simulink model "RotorTune_ver3f"  (R2024a)
settings: Solver=FixedStepAuto  StartTime=0.0  StopTime=Inf  FixedStep=SampleTs  RelTol=1e-3  EnableMultiTasking=on
values from neighbouring files (symbols this model uses):
  A = [0, 1 ... (first row only)    [linearisze_lqr_design.m]
undefined symbols (not defined in the file or in its folder): ControlTs, ctrlDen, ctrlNum, Den, Down, EncBias, EncRes, fdbkctrl, fdbkopt, GPTRIP1SEL, Num, SampleTs, SimTime, StartTime, StepMagnitude, T_L, TZ1, Up, VelRes
libraries: simulink x3, c2837xDlib x1, c2802xlib x1, c280xlib x1
settings Model: SimulationMode=external  ExtModeTrigDuration=8  Creator=Student  LastModifiedBy=MAELAB_05
settings OptimizationCC: DefaultUnderspecifiedDataType=single  EnhancedBackFolding=on  PassReuseOutputArgsAs=Individual arguments  MaxStackSize=1024  OptimizeBlockOrder=speed  DifferentSizesBufferReuse=on  OptimizationCustomize=off  DenormalBehavior=FlushToZero  EfficientTunableParamExpr=on
settings DebuggingCC: ParameterTunabilityLossMsg=error
settings HardwareCC: ProdBitPerChar=16  ProdBitPerInt=16  ProdBitPerPointer=32  ProdBitPerSizeT=32  ProdBitPerPtrDiffT=32  ProdLargestAtomicInteger=Integer  ProdLargestAtomicFloat=None  ProdWordSize=16  ProdLongLongMode=on  ProdHWDeviceType=Texas Instruments->C2000
settings ModelReferenceCC: ModelReferenceNumInstancesAllowed=Single
settings SFSimCC: MATLABDynamicMemAlloc=off
settings RTWCC: Description=Embedded Coder  SystemTargetFile=ert.tlc  HardwareBoard=TI Delfino F28379D LaunchPad  TemplateMakefile=ert_default_tmf  Toolchain=Texas Instruments Code Composer Studio (C2000)  CodeProfilingSaveOptions=MetricsOnly  GPUComputeCapability=3.5
settings CodeAppCC: ForceParamTrailComments=on  IgnoreCustomStorageClasses=off  OperatorAnnotations=on  SimulinkDataObjDesc=on  SFDataObjDesc=on  InsertBlockDesc=on
settings ERTTargetCC: CodeReplacementLibrary=TI C28x  ExtMode=on  ExtModeTransport=4  ExtModeStaticAlloc=on  ExtModeAutomaticAllocSize=off  ExtModeStaticAllocSize=10000  ExtModeMexFile=ext_xcp  ExtModeMexArgs=1 4 5000000  ExtModeIntrfLevel=Level2 - Open

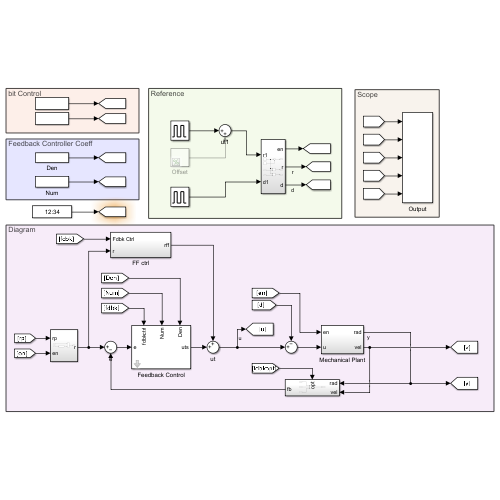
[thumbnail: Simulink's stored preview of the top-level diagram]
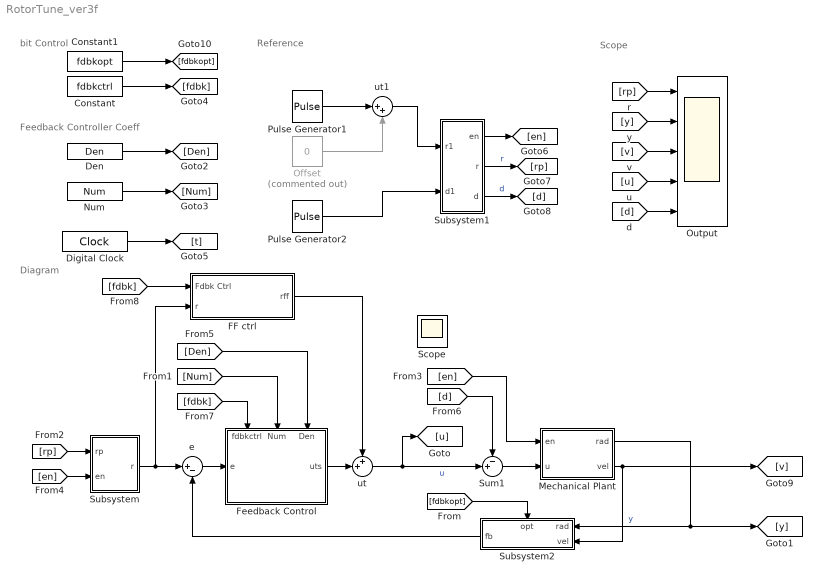
== system RotorTune_ver3f ==
  note: Diagram
  note: Scope
  note: Reference
  note: bit Control
  note: Feedback Controller Coeff
  Constant : Constant  Value=fdbkctrl  OutDataTypeStr=double  SampleTime=SampleTs
  Constant1 : Constant  Value=fdbkopt  OutDataTypeStr=double  SampleTime=SampleTs
  Den : Constant  Value=Den  SampleTime=ControlTs
  Digital Clock : DigitalClock  SampleTime=SampleTs
  FF ctrl : Subsystem
  Feedback Control : Subsystem  mask(Discrete Time Controller){}
      mask help: Discrete IIR filter with output saturation. Please write the controller in filter form before writing the numerator and denominator coefficients.
      settings: PortSchema="{\"entries\":[{\"content\":{\"sides\":[{\"content\":{\"connectorIds\":[\"In1\"]},\"type\":\"ConnectorPlacement.EquallySpacedRectSide\",\"uuid\":\"e0eb88a8-3f62-4736-a83e-fbf139955186\"},{\"content\":{\"connectorIds\":[\"Out1\"],\"side\":\"RIGHT\"},\"type\":\"ConnectorPlacement.EquallySpacedRectSide\",\"uuid\":\"655529f7-d729-4d0c-b17c-6f52c7004a6d\"},{\"content\":{\"connectorIds\":[\"In2\",\"In3\",\"In4\"],\"side\":\"TOP\"},\"type\":\"ConnectorPlacement.EquallySpacedRectSide\",\"uuid\":\"a879eb77-4166-453f-a794-1fc287420031\"},{\"content\":{\"connectorIds\":[],\"side\":\"BOTTOM\"},\"type\":\"ConnectorPlacement.EquallySpacedRectSide\",\"uuid\":\"f5f0df5c-bd43-42ec-91f5-1b4d11260522\"}]},\"type\":\"ConnectorPlacement.EquallySpacedConnector\",\"uuid\":\"5f5b86c4-0571-4a61-ae4f-21c2576f152a\"}],\"packageUris\":[\"http://schema.mathworks.com/mf0/Connector/R2020b\"],\"version\":\"1.0\"}"
  Mechanical Plant : Subsystem
  Num : Constant  Value=Num  SampleTime=ControlTs
  Offset : Constant  Commented=on  Value=0
  Output : Scope  NumInputPorts=5
  Pulse Generator1 : DiscretePulseGenerator  PulseType=Time based  Amplitude=StepMagnitude  Period=10  PulseWidth=50
  Pulse Generator2 : DiscretePulseGenerator  PulseType=Time based  Amplitude=T_L*fdbkctrl  Period=10  PulseWidth=50  PhaseDelay=1
  Subsystem : Subsystem
  Subsystem1 : Subsystem
  Subsystem2 : Subsystem
      settings: PortSchema="{\"entries\":[{\"content\":{\"sides\":[{\"content\":{\"connectorIds\":[\"Out1\"]},\"type\":\"ConnectorPlacement.EquallySpacedRectSide\",\"uuid\":\"4f8a58ab-8b77-4548-a5e4-8c342b5af4de\"},{\"content\":{\"connectorIds\":[\"In2\",\"In3\"],\"side\":\"RIGHT\"},\"type\":\"ConnectorPlacement.EquallySpacedRectSide\",\"uuid\":\"f569d0f3-df36-4b5a-9df6-29756aab0033\"},{\"content\":{\"connectorIds\":[\"In1\"],\"side\":\"TOP\"},\"type\":\"ConnectorPlacement.EquallySpacedRectSide\",\"uuid\":\"c4523680-dffb-4dca-b5af-4725fc2c115b\"}]},\"type\":\"ConnectorPlacement.EquallySpacedConnector\",\"uuid\":\"6d4037b4-5141-4a52-bd71-8d22041459e1\"}],\"packageUris\":[\"http://schema.mathworks.com/mf0/Connector/R2020b\"],\"version\":\"1.0\"}"
  Sum1 : Sum  Inputs=-+|
  e : Sum  Inputs=|+-
  ut : Sum  Inputs=++|
  ut1 : Sum  Inputs=|++
  Scope : Scope
  wires:
  [en] -> Mechanical Plant/1(en)
  Feedback Control/1(uts) -> ut/2
  [rp] -> Subsystem/1(rp)
  [en] -> Subsystem/2(en)
  Subsystem/1(r) -> e/1, FF ctrl/2(r)
  FF ctrl/1(rff) -> ut/1
  e/1 -> Feedback Control/1(e)
  [fdbk] -> Feedback Control/2(fdbkctrl)
  Den/1 -> [Den]
  Num/1 -> [Num]
  [Den] -> Feedback Control/4(Den)
  Constant/1 -> [fdbk]
  ut/1 -> Sum1/2, [u]  "u"
  [d] -> Sum1/1
  Sum1/1 -> Mechanical Plant/2(u)
  Subsystem1/1(en) -> [en]
  Subsystem1/2(r) -> [rp]  "r"
  Subsystem1/3(d) -> [d]  "d"
  [rp] -> Output/1
  [y] -> Output/2
  Mechanical Plant/2(vel) -> Subsystem2/3(vel), [v]
  [v] -> Output/3
  [u] -> Output/4
  [d] -> Output/5
  ut1/1 -> Subsystem1/1(r1)
  Pulse Generator1/1 -> ut1/1
  Offset/1 -> ut1/2
  Digital Clock/1 -> [t]
  [Num] -> Feedback Control/3(Num)
  [fdbk] -> FF ctrl/1(Fdbk Ctrl)
  Constant1/1 -> [fdbkopt]
  [fdbkopt] -> Subsystem2/1(opt)
  Subsystem2/1(fb) -> e/2
  Pulse Generator2/1 -> Subsystem1/2(d1)
  Mechanical Plant/1(rad) -> [y], Subsystem2/2(rad)  "y"

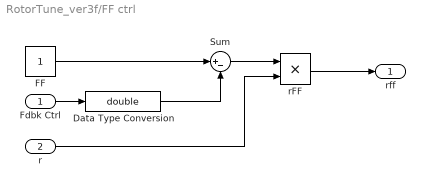
== system RotorTune_ver3f/FF ctrl ==
  Fdbk Ctrl : Inport
  r : Inport  Port=2
  Data Type Conversion : DataTypeConversion  OutDataTypeStr=double  SaturateOnIntegerOverflow=off  RndMeth=Floor
  FF : Constant  SampleTime=SampleTs
  Sum : Sum  Inputs=|+-
  rFF : Product
  rff : Outport
  wires:
  Sum/1 -> rFF/1
  FF/1 -> Sum/1
  Fdbk Ctrl/1 -> Data Type Conversion/1
  rFF/1 -> rff/1
  r/1 -> rFF/2
  Data Type Conversion/1 -> Sum/2

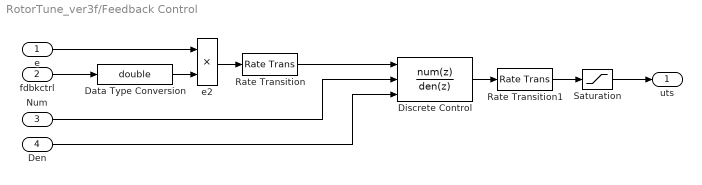
== system RotorTune_ver3f/Feedback Control ==
  e : Inport
  fdbkctrl : Inport  Port=2
  Num : Inport  Port=3
  Den : Inport  Port=4
  Data Type Conversion : DataTypeConversion  OutDataTypeStr=double  SaturateOnIntegerOverflow=off  RndMeth=Floor
  Discrete Control : DiscreteFilter  NumeratorSource=Input port  Numerator=ctrlNum  DenominatorSource=Input port  Denominator=ctrlDen  SampleTime=ControlTs  a0EqualsOne=on
      settings: InputPortMap=u0,p1,p3
  Rate Transition : RateTransition  OutPortSampleTime=ControlTs
  Rate Transition1 : RateTransition  OutPortSampleTime=SampleTs
  Saturation : Saturate  UpperLimit=1  LowerLimit=-1
  e2 : Product
  uts : Outport
  wires:
  Saturation/1 -> uts/1
  Num/1 -> Discrete Control/2
  Den/1 -> Discrete Control/3
  Rate Transition/1 -> Discrete Control/1
  Discrete Control/1 -> Rate Transition1/1
  Rate Transition1/1 -> Saturation/1
  e2/1 -> Rate Transition/1
  e/1 -> e2/1
  Data Type Conversion/1 -> e2/2
  fdbkctrl/1 -> Data Type Conversion/1

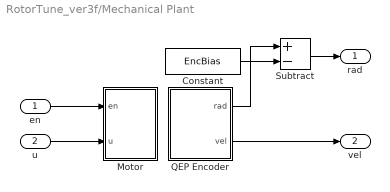
== system RotorTune_ver3f/Mechanical Plant ==
  en : Inport
  u : Inport  Port=2
  Constant : Constant  Value=EncBias  SampleTime=SampleTs
  Motor : Subsystem  mask(Maxon Motor){}
      mask help: Input duty cycle to 20 kHz carrier frequency PWM brushed dc dual h-bridge.
  QEP Encoder : Subsystem  mask(Incremental Quadrature Encoder){}
      mask help: Quadrature Encoder for DC brushed motor, single-ended channel.
  Subtract : Sum  Inputs=+-
  rad : Outport
  vel : Outport  Port=2
  wires:
  u/1 -> Motor/2(u)
  QEP Encoder/1(rad) -> Subtract/1
  en/1 -> Motor/1(en)
  QEP Encoder/2(vel) -> vel/1
  Constant/1 -> Subtract/2
  Subtract/1 -> rad/1

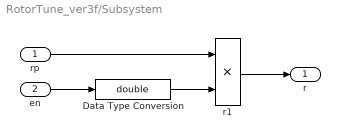
== system RotorTune_ver3f/Subsystem ==
  rp : Inport
  en : Inport  Port=2
  Data Type Conversion : DataTypeConversion  OutDataTypeStr=double  SaturateOnIntegerOverflow=off  RndMeth=Floor
  r1 : Product
  r : Outport
  wires:
  en/1 -> Data Type Conversion/1
  rp/1 -> r1/1
  r1/1 -> r/1
  Data Type Conversion/1 -> r1/2

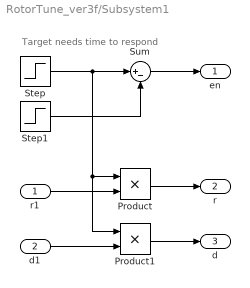
== system RotorTune_ver3f/Subsystem1 ==
  note: Target needs time to respond
  r1 : Inport
  d1 : Inport  Port=2
  Product : Product
  Product1 : Product
  Step : Step  Time=StartTime  SampleTime=SampleTs
  Step1 : Step  Time=SimTime-5  SampleTime=SampleTs
  Sum : Sum  Inputs=|+-
  en : Outport
  r : Outport  Port=2
  d : Outport  Port=3
  wires:
  Step1/1 -> Sum/2
  Step/1 -> Product1/1, Product/1, Sum/1
  Sum/1 -> en/1
  r1/1 -> Product/2
  Product/1 -> r/1
  d1/1 -> Product1/2
  Product1/1 -> d/1

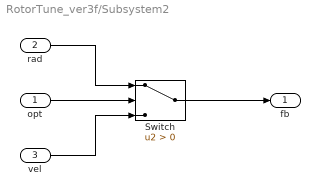
== system RotorTune_ver3f/Subsystem2 ==
  opt : Inport
  rad : Inport  Port=2
  vel : Inport  Port=3
  Switch : Switch  Criteria=u2 > Threshold  SaturateOnIntegerOverflow=off  InputSameDT=off
  fb : Outport
  wires:
  rad/1 -> Switch/1
  opt/1 -> Switch/2
  Switch/1 -> fb/1
  vel/1 -> Switch/3

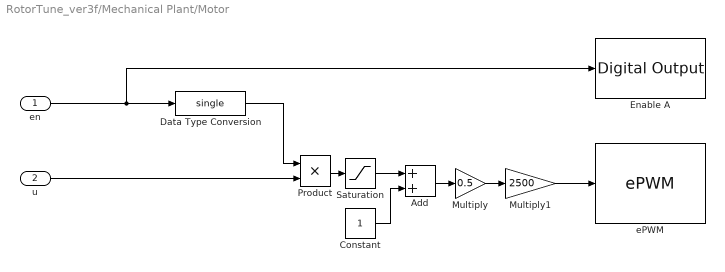
== system RotorTune_ver3f/Mechanical Plant/Motor ==
  en : Inport
  u : Inport  Port=2
  Add : Sum
  Constant : Constant  SampleTime=-1
  Data Type Conversion : DataTypeConversion  OutDataTypeStr=single  SaturateOnIntegerOverflow=off  RndMeth=Floor
  Enable A : c2837xDlib/Digital Output  GPIO_Number=GPIO56~GPIO63  GPIO_Bit0=off  GPIO_BIT0_Toggle=off  GPIO_Bit1=off  GPIO_BIT1_Toggle=off  GPIO_Bit2=off  GPIO_BIT2_Toggle=off  GPIO_Bit3=off  GPIO_BIT3_Toggle=off  GPIO_Bit4=off  GPIO_BIT4_Toggle=off  GPIO_Bit5=on  GPIO_BIT5_Toggle=off  GPIO_Bit6=off  GPIO_BIT6_Toggle=off  GPIO_Bit7=off  GPIO_BIT7_Toggle=off
  Multiply : Gain  Gain=0.5
  Multiply1 : Gain  Gain=2500
  Product : Product
  Saturation : Saturate  UpperLimit=1  LowerLimit=-1
  ePWM : c2802xlib/ePWM  PwmType=C2000_Type4  useModule=ePWM1  ePWMxLINKTBPRD=Not Linked  periodUnits=Clock cycles  timerSource=Specify via dialog  timerPeriod_clk=2500  timerPeriod_sec=0.0001  tbshadow=Counter equals to zero  countingMode=Up-Down  phaseActiveEnable=Disable  phaseDirection=Count down after sync  phaseActive=0  synchronizationEnable=off  dcaevt1Sync=off  dcbevt1Sync=off  synchronizationOption=Disable  dcbevt1SyncOut=off  dcaevt1SyncOut=off  cmpdSyncOut=off  cmpcSyncOut=off  cmpbSyncOut=off  zeroSyncOut=off  swfSyncOut=off  perSynchronizationOption=Counter equals to period (CTR=PRD)  clockPrescale=1  HSclockPrescale=1  enswap=off  ePWMxAStatus=on  ePWMxAactionLogic1=Set  ePWMxAactionLogic2=Clear  ePWMxAactionLogic3=Clear  ePWMxAactionLogic4=Set  ePWMxAactionLogic5=Do nothing  ePWMxAactionLogic6=Do nothing  ePWMxACSFenable=off  ePWMxACSFvalue=Forcing disable  ePWMxASFreload=Zero  ePWMxBStatus=on  ePWMxBactionLogic1=Do nothing  ePWMxBactionLogic2=Do nothing  ePWMxBactionLogic3=Set  ePWMxBactionLogic4=Clear  ePWMxBactionLogic5=Do nothing  ePWMxBactionLogic6=Do nothing  ePWMxBCSFenable=off  ePWMxBCSFvalue=Forcing disable  ePWMxBSFreload=Zero  ePWNxBOutWay=off  ePWMxLINKCMPA=Not Linked  CMPAUnits=Clock cycles  CMPASource=Input port  CMPAValue_per=50  CMPAValue_clk=1250  enCMPAshadow=Counter equals to zero (CTR=Zero)  ePWMxLINKCMPB=Not Linked  CMPBUnits=Clock cycles  CMPBSource=Specify via dialog  CMPBValue_per=50  CMPBValue_clk=1250  enCMPBshadow=Counter equals to zero (CTR=Zero)  ePWMxLINKCMPC=Not Linked  CMPCUnits=Clock cycles  CMPCSource=Specify via dialog  CMPCValue_per=50  CMPCValue_clk=32000  enCMPCshadow=Counter equals to zero (CTR=Zero)  ePWMxLINKCMPD=Not Linked  CMPDUnits=Clock cycles  CMPDSource=Specify via dialog  CMPDValue_per=50  CMPDValue_clk=32000  enCMPDshadow=Counter equals to zero (CTR=Zero)  enableDBePWMxA=off  enableDBePWMxB=off  enhalfcycle=off  DBpolarity=Active high (AH)  DBedgeDelay=Positive  DBSource_ePWMxA=ePWMxA  DBSource_ePWMxB=ePWMxA  DBPeriodUnits=Clock cycles  DBperiodSource=Specify via dialog  REDperiod=0  FEDperiod=0  REDperiod_sec=0  FEDperiod_sec=0  LoadModeDBRED=Immediate without using shadow  LoadModeDBFED=Immediate without using shadow  adcstartModuleA=off  adcrequestEventA=First event  adcstartEventA=Digital Compare Module A Event 1 start of conversion (DCAEVT1.soc)  adcstartEventA_type2=Counter equals to zero (CTR=Zero)  adcstartModuleB=off  adcrequestEventB=First event  adcstartEventB=Counter equals to zero (CTR=Zero)  adcstartEventB_type2=Counter equals to zero (CTR=Zero)  intEn=off  intPrd=First event  intSel=Counter equals to zero (CTR=Zero)  intSel_type2=Counter equals to zero (CTR=Zero)  hrpe=off  enHRPWM=off  HRPWM_LoadMode=Counter equals to period (CTR=PRD)  HRPWM_CTLMode=Duty or Period control mode  HRPWM_EDGMode=Both edge  hrpeb=off  enHRPWMB=off  HRPWM_LoadModeB=Counter equals to zero (CTR=ZERO)  HRPWM_CTLModeB=Duty or Period control mode  HRPWM_EDGModeB=Both edge  enHRDBRED=off  enHRDBFED=off  enSFO=on  enautoconv=on  chopperEnable=off  chopperFrequency=1  chopperFirstwidth=1  chopperDuty=12.5%  tripZonesource=Specify via dialog  tzselOSHT1=off  tzselOSHT2=off  tzselOSHT3=off  tzselOSHT4=off  tzselOSHT5=off  tzselOSHT6=off  tzselOSHDCAEV1=off  tzselOSHDCBEV1=off  tzselCBC1=off  tzselCBC2=off  tzselCBC3=off  tzselCBC4=off  tzselCBC5=off  tzselCBC6=off  tzselCBCDCAEV2=off  tzselCBCDCBEV2=off  enTzOstIntr=off  enTzCbcIntr=off  enTzDCAEVT1Intr=off  enTzDCAEVT2Intr=off  enTzDCBEVT1Intr=off  enTzDCBEVT2Intr=off  tzclrCBCLatch=Counter equals to zero (CTR=Zero)  ePWMxAforced=No action  ePWMxBforced=No action  DCAEVT1forced=No action  DCBEVT1forced=No action  DCAEVT2forced=No action  DCBEVT2forced=No action  dcah=Trip Zone 1 input (TZ1)  dcal=Trip Zone 2 input (TZ2)  dcbh=Trip Zone 1 input (TZ1)  dcbl=Trip Zone 2 input (TZ2)  dcah_type2=GPTRIP1SEL/(TZ1)  dcal_type2=GPTRIP1SEL/(TZ1)  dcbh_type2=GPTRIP1SEL/(TZ1)  dcbl_type2=GPTRIP1SEL/(TZ1)  gendcaevt1=Event disabled  gendcaevt2=Event disabled  gendcbevt1=Event disabled  gendcbevt2=Event disabled  dcaevt1src=DCAEVT1 with sync  dcaevt2src=DCAEVT2 with sync  dcbevt1src=DCBEVT1 with sync  dcbevt2src=DCBEVT2 with sync  pulsesel=Counter equals to zero (CTR=Zero)  blankinv=off  blankoffset=0  blankwidth=0  evsrcsel=Filtered version of DCAEVT1 (DCAEVT1FILT)  encape=off
      settings: LibrarySourceBlock=c2837xDlib/ePWM
  wires:
  Multiply/1 -> Multiply1/1
  Add/1 -> Multiply/1
  Multiply1/1 -> ePWM/1
  Constant/1 -> Add/2
  Saturation/1 -> Add/1
  Product/1 -> Saturation/1
  u/1 -> Product/2
  Data Type Conversion/1 -> Product/1
  en/1 -> Enable A/1, Data Type Conversion/1

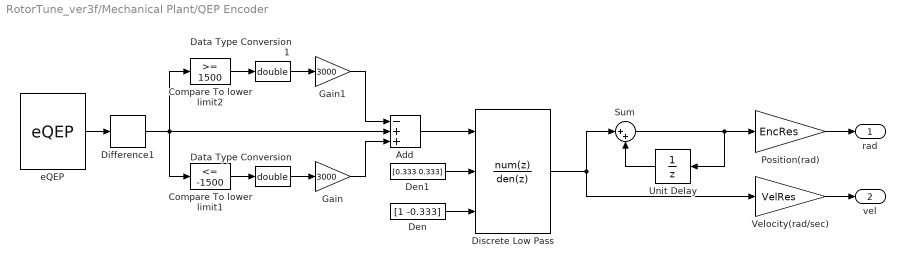
== system RotorTune_ver3f/Mechanical Plant/QEP Encoder ==
  Add : Sum  Inputs=-++
  Compare To lower limit1 : simulink/Logic and Bit Operations/Compare To Constant  relop=<=  const=-1500  OutDataTypeStr=boolean
  Compare To lower limit2 : simulink/Logic and Bit Operations/Compare To Constant  relop=>=  const=1500  OutDataTypeStr=boolean
  Data Type Conversion : DataTypeConversion  OutDataTypeStr=double  SaturateOnIntegerOverflow=off  RndMeth=Floor
  Data Type Conversion1 : DataTypeConversion  OutDataTypeStr=double  SaturateOnIntegerOverflow=off  RndMeth=Floor
  Den : Constant  Value=[1 -0.333]  SampleTime=SampleTs
  Den1 : Constant  Value=[0.333 0.333]  SampleTime=SampleTs
  Difference1 : simulink/Discrete/Difference  ICPrevInput=0.0  OutMin=[]  OutMax=[]  OutDataType=fixdt(1, 16)  OutScaling=2^-10  DoSatur=off
  Discrete Low Pass : DiscreteFilter  NumeratorSource=Input port  Numerator=ctrlNum  DenominatorSource=Input port  Denominator=ctrlDen  SampleTime=SampleTs  a0EqualsOne=on
      settings: InputPortMap=u0,p1,p3
  Gain : Gain  Gain=3000
  Gain1 : Gain  Gain=3000
  Position(rad) : Gain  Gain=EncRes
  Sum : Sum  Inputs=|++
  Unit Delay : UnitDelay  SampleTime=SampleTs  HasFrameUpgradeWarning=on
  Velocity(rad/sec) : Gain  Gain=VelRes
  eQEP : c280xlib/eQEP  useModule=eQEP1  pcInputmode=Quadrature-count  externalClockrate=2x resolution: Count the rising/falling edge  swapPolarityselection=Clockwise  qdfOutputport=off  qapPolarityselection=off  qbpPolarityselection=off  qipPolarityselection=off  qspPolarityselection=off  igatePolarityselection=off  sampleTime=SampleTs  pcOutputport=on  pcMaximumvalue=3000  indexInitializationcheck=off  indexInitializationevent=Rising edge  strobeInitializationcheck=off  strobeInitializationevent=Rising edge  softwareInitializationcheck=on  softwareInitializationsource=Set to init value at start up  softwareInitializationmode=on  pcInitialvalue=1500  pcResetmode=Reset on an index event  ieloutputport=off  indexEventlatch=Rising edge  seloutputport=off  strobeEventlatch=Rising edge  pcefOutputport=off  enableEqepcapture=off  qctmrOutputport=off  qcprdOutputport=on  captureTimerprescaler=128  upEventprescaler=1  overflowErrorflag=off  directionErrorflag=off  captureTimerposition=On position counter read  unitTimerperiod=100000000  captureTimerlatch=off  capturePeriodlatch=off  positionCounterlatch=off  soenPolarityselection=off  spselPolarityselection=Index pin is used for sync output  compareValuesource=Specify via dialog  shadowMode=Load on QPOSCNT=0  compareValue=4294967295  syncOutputwidth=1  polaritySyncoutput=Active high  watchdogEnable=off  watchdogTimer=65535  outport1Datatype=auto  outport2Datatype=auto  outport3Datatype=auto  outport4Datatype=auto  outport5Datatype=auto  outport6Datatype=auto  outport7Datatype=auto  outport8Datatype=auto  outport9Datatype=auto  outport10Datatype=auto  outport11Datatype=auto  outport12Datatype=auto  eqepinterrupt_pce=off  eqepinterrupt_qpe=off  eqepinterrupt_qdc=off  eqepinterrupt_wto=off  eqepinterrupt_pcu=off  eqepinterrupt_pco=off  eqepinterrupt_pcr=off  eqepinterrupt_pcm=off  eqepinterrupt_sel=off  eqepinterrupt_iel=off  eqepinterrupt_uto=off  pheOutputport=off  watchdogOutputport=off  outport13Datatype=auto  outport14Datatype=auto
      settings: LibrarySourceBlock=c2837xDlib/eQEP
  rad : Outport
  vel : Outport  Port=2
  wires:
  Discrete Low Pass/1 -> Velocity(rad/sec)/1, Sum/1
  Velocity(rad/sec)/1 -> vel/1
  Compare To lower limit1/1 -> Data Type Conversion/1
  Data Type Conversion/1 -> Gain/1
  Data Type Conversion1/1 -> Gain1/1
  Compare To lower limit2/1 -> Data Type Conversion1/1
  Gain1/1 -> Add/1
  eQEP/1 -> Difference1/1
  Gain/1 -> Add/3
  Difference1/1 -> Compare To lower limit2/1, Compare To lower limit1/1, Add/2
  Sum/1 -> Position(rad)/1, Unit Delay/1
  Unit Delay/1 -> Sum/2
  Position(rad)/1 -> rad/1
  Add/1 -> Discrete Low Pass/1
  Den/1 -> Discrete Low Pass/3
  Den1/1 -> Discrete Low Pass/2
